simulink model "oppg2_f"  (R2020b)
settings: Solver=VariableStepAuto  StartTime=0.0  StopTime=100.0  RelTol=1e-3
values from neighbouring files (symbols this model uses):
  A = [   -0.322,     0.052,      0.028,      -1.12,      0.002 ... (first row only)    [linear_aircraft_model_constants.m]
  B = [   0 ... (first row only)    [linear_aircraft_model_constants.m]
  C = [   1,  0,  0,  0,  0 ... (first row only)    [linear_aircraft_model_constants.m]
  d = deg2rad(1.5)    [linear_aircraft_model_constants.m]
  delta_a_max = delta_a_max    [linear_aircraft_model_constants.m]
  g = 9.81    [linear_aircraft_model_constants.m]
  k_i_chi = omega_n_chi^2*V_g/g    [linear_aircraft_model_constants.m]
  k_i_phi = 0    [linear_aircraft_model_constants.m]    (also in oppg2.m = k_i_min + i*res)
  k_p_chi = 2*zeta_chi*omega_n_chi*V_g/g    [linear_aircraft_model_constants.m]
  k_p_phi = delta_a_max/e_phi_max * sign(a_phi2)    [linear_aircraft_model_constants.m]
  V_g = 580/3.6    (= 161.111111111)    [linear_aircraft_model_constants.m]
settings Model: Creator=danie  LastModifiedBy=simengangstad

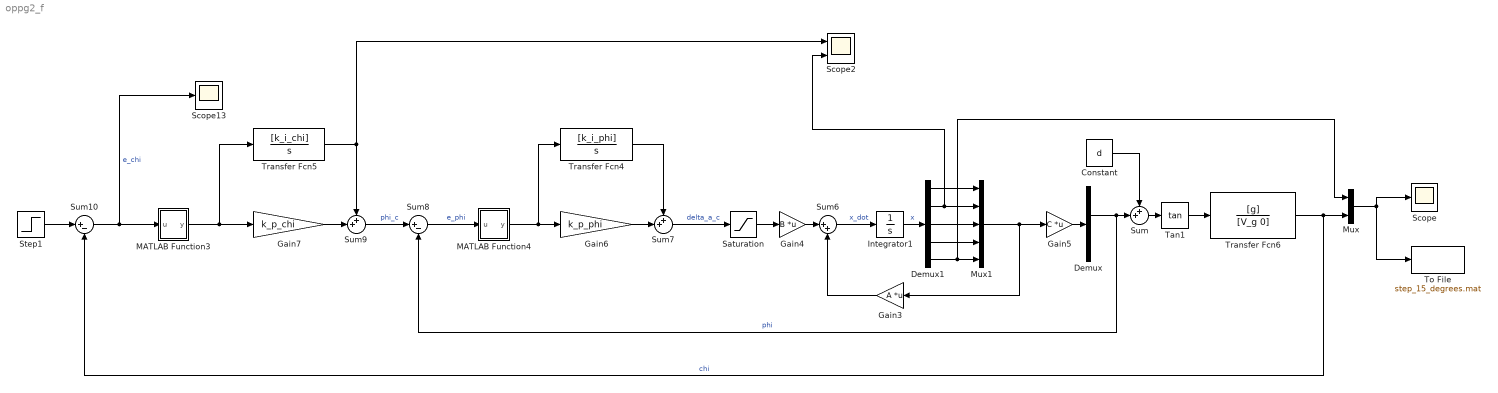
== system oppg2_f ==
  Constant : Constant  Value=d
  Demux : Demux
  Demux1 : Demux  Outputs=5
  Gain3 : Gain  Gain=A  Multiplication=Matrix(K*u)
  Gain4 : Gain  Gain=B  Multiplication=Matrix(K*u)
  Gain5 : Gain  Gain=C  Multiplication=Matrix(K*u)
  Gain6 : Gain  Gain=k_p_phi
  Gain7 : Gain  Gain=k_p_chi
  Integrator1 : Integrator
  MATLAB Function3 : MATLAB Function  TreatAsAtomicUnit=on
  MATLAB Function4 : MATLAB Function  TreatAsAtomicUnit=on
  Mux : Mux  Inputs=2
  Mux1 : Mux  Inputs=5
  Saturation : Saturate  UpperLimit=delta_a_max  LowerLimit=-delta_a_max
  Scope : Scope
  Scope13 : Scope
  Scope2 : Scope  NumInputPorts=2
  Step1 : Step  Time=5  After=15*pi/180  SampleTime=0
  Sum : Sum  Inputs=++|
  Sum10 : Sum  Inputs=|+-
  Sum6 : Sum  Inputs=|++
  Sum7 : Sum  Inputs=++|
  Sum8 : Sum  Inputs=|+-
  Sum9 : Sum  Inputs=++|
  Tan1 : Trigonometry  Operator=tan
  To File : ToFile  Filename=step_15_degrees.mat
  Transfer Fcn4 : TransferFcn  Numerator=[k_i_phi]  Denominator=[1 0]
  Transfer Fcn5 : TransferFcn  Numerator=[k_i_chi]  Denominator=[1 0]
  Transfer Fcn6 : TransferFcn  Numerator=[g]  Denominator=[V_g 0]
  wires:
  Integrator1/1 -> Demux1/1  "x"
  Gain4/1 -> Sum6/1
  Sum6/1 -> Integrator1/1  "x_dot"
  Gain3/1 -> Sum6/2
  Gain5/1 -> Demux/1
  MATLAB Function3/1(y) -> Transfer Fcn5/1, Gain7/1
  Sum9/1 -> Sum8/1  "phi_c"
  Gain7/1 -> Sum9/2
  Transfer Fcn5/1 -> Scope2/1, Sum9/1
  MATLAB Function4/1(y) -> Transfer Fcn4/1, Gain6/1
  Gain6/1 -> Sum7/2
  Sum8/1 -> MATLAB Function4/1(u)  "e_phi"
  Sum10/1 -> MATLAB Function3/1(u), Scope13/1  "e_chi"
  Tan1/1 -> Transfer Fcn6/1
  Transfer Fcn6/1 -> Sum10/2, Mux/2  "chi"
  Step1/1 -> Sum10/1
  Mux/1 -> Scope/1, To File/1
  Demux1/5 -> Mux1/5, Mux/1
  Demux1/4 -> Mux1/4
  Demux1/3 -> Mux1/3
  Demux1/1 -> Mux1/1
  Mux1/1 -> Gain5/1, Gain3/1
  Sum7/1 -> Saturation/1  "delta_a_c"
  Saturation/1 -> Gain4/1
  Demux/2 -> Sum/2, Sum8/2  "phi"
  Sum/1 -> Tan1/1
  Constant/1 -> Sum/1
  Transfer Fcn4/1 -> Sum7/1
  Demux1/2 -> Scope2/2, Mux1/2

== matlab function oppg2_f/MATLAB Function4 ==
  data: u input; y output
function y = fcn(u)

y = angdiff(0,u);

== matlab function oppg2_f/MATLAB Function3 ==
  data: u input; y output
function y = fcn(u)

y = angdiff(0,u);
